simulink model "PoleZeroAndFreqResp"  (R2022b)
settings: Solver=VariableStepAuto  StartTime=0.0  StopTime=10.0  MaxStep=1e-5  MinStep=1e-6  RelTol=1e-3
settings Model: Creator=yeyi5  LastModifiedBy=yeyi5

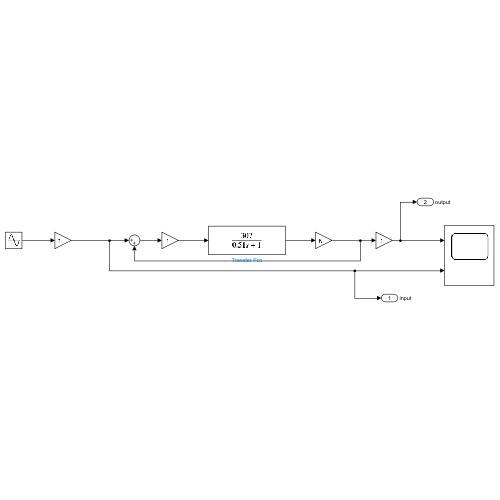
[thumbnail: Simulink's stored preview of the top-level diagram]
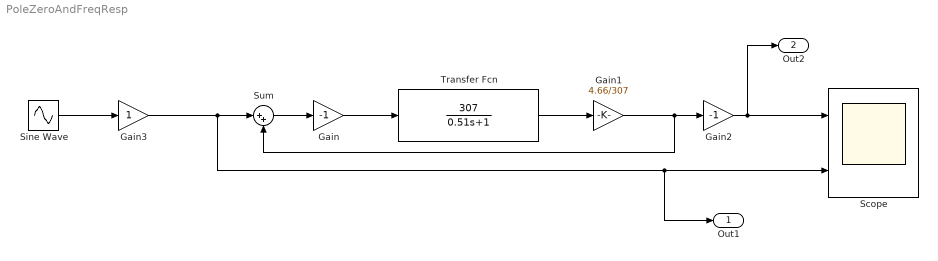
== system PoleZeroAndFreqResp ==
  Gain : Gain  Gain=-1
  Gain1 : Gain  Gain=4.66/307
  Gain2 : Gain  Gain=-1
  Gain3 : Gain
  Scope : Scope  NumInputPorts=2
  Sine Wave : Sin  SampleTime=0
  Sum : Sum  Inputs=|++
  Transfer Fcn : TransferFcn  Numerator=[307]  Denominator=[0.51 1]
  Out1 : Outport  SignalName=input
  Out2 : Outport  Port=2  SignalName=output
  wires:
  Sine Wave/1 -> Gain3/1
  Gain1/1 -> Sum/2, Gain2/1
  Gain/1 -> Transfer Fcn/1
  Transfer Fcn/1 -> Gain1/1
  Gain2/1 -> Out2/1, Scope/1
  Sum/1 -> Gain/1
  Gain3/1 -> Out1/1, Scope/2, Sum/1
